simulink model "B_LazoCerrado_PI"  (R2017a)
settings: Solver=FixedStepAuto  StartTime=0.0  StopTime=inf  RelTol=1e-3  EnableMultiTasking=on
libraries: arduinolib x2, simulink x1
settings Model: SimulationMode=external  ExtModeTrigDuration=2  Creator=pablo  LastModifiedBy=pablo
settings OptimizationCC: PassReuseOutputArgsAs=Individual arguments  MaxStackSize=64
settings DebuggingCC: ParameterTunabilityLossMsg=error
settings HardwareCC: ProdBitPerInt=16  ProdBitPerPointer=16  ProdBitPerSizeT=16  ProdBitPerPtrDiffT=16  ProdLargestAtomicFloat=None  ProdWordSize=8  ProdHWDeviceType=Atmel->AVR
settings SFSimCC: MATLABDynamicMemAlloc=off
settings RTWCC: SystemTargetFile=ert.tlc  HardwareBoard=Arduino Uno  TLCOptions=-aInlineSetEventsForThisBaseRateFcn=TLC_FALSE -aSuppressMultiTaskScheduler=TLC_FALSE -aRateBasedStepFcn=1  TemplateMakefile=ert_default_tmf  Description=Embedded Coder  GenerateReport=on  Toolchain=Arduino AVR  BuildConfiguration=Faster Runs  IncludeHyperlinkInReport=on  LaunchReport=on  GenerateTraceInfo=on  GenerateTraceReport=on  GenerateTraceReportSl=on  GenerateTraceReportSf=on  GenerateTraceReportEml=on
settings CodeAppCC: ForceParamTrailComments=on  IgnoreCustomStorageClasses=off  OperatorAnnotations=on  SimulinkDataObjDesc=on  SFDataObjDesc=on  MATLABFcnDesc=on  InsertBlockDesc=on  MATLABSourceComments=on
settings ERTTargetCC: SupportContinuousTime=on  SupportVariableSizeSignals=on

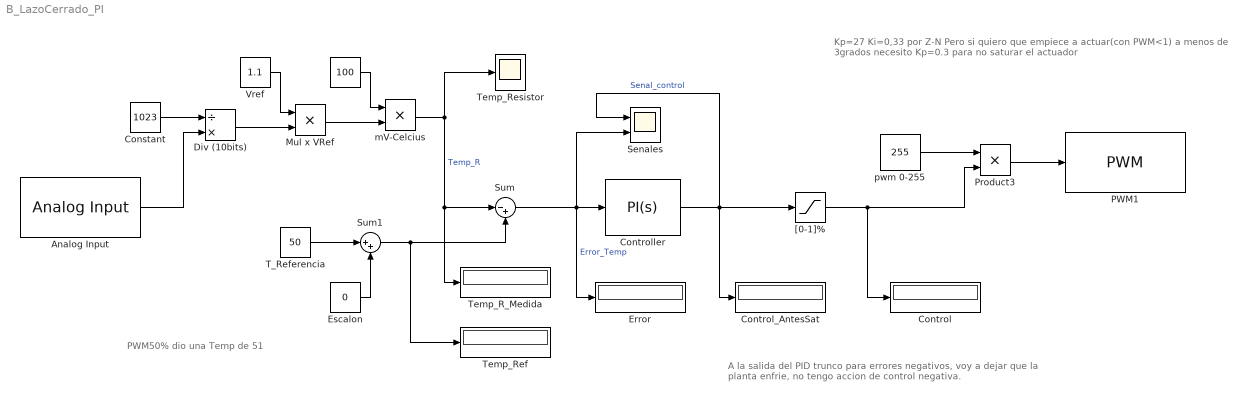
== system B_LazoCerrado_PI ==
  note: PWM50% dio una Temp de 51
  note: Kp=27 Ki=0,33 por Z-N
      | Pero si quiero que empiece a actuar(con PWM<1)
      | a menos de 3grados necesito Kp=0.3
      | para no saturar el actuador
  note: A la salida del PID trunco para errores negativos,
      | voy a dejar que la planta enfrie, no tengo accion de control negativa.
  " " : Constant  Value=100
  " Controller" : simulink/Continuous/PID Controller  Controller=PI  TimeDomain=Continuous-time  SampleTime=-1  IntegratorMethod=Forward Euler  FilterMethod=Forward Euler  Form=Parallel  UseFilter=on  ControllerParametersSource=internal  P=0.1  I=0.0001  D=0  N=100  InitialConditionSource=internal  InitialConditionForIntegrator=0  InitialConditionForFilter=0  ExternalReset=none  LimitOutput=on  UpperSaturationLimit=inf  LowerSaturationLimit=0  LinearizeAsGain=on  AntiWindupMode=none  Kb=1  TrackingMode=off  Kt=1  PParamMin=[]  PParamMax=[]  IParamMin=[]  IParamMax=[]  DParamMin=[]  DParamMax=[]  NParamMin=[]  NParamMax=[]  KbParamMin=[]  KbParamMax=[]  KtParamMin=[]  KtParamMax=[]  POutMin=[]  POutMax=[]  IOutMin=[]  IOutMax=[]  DOutMin=[]  DOutMax=[]  NOutMin=[]  NOutMax=[]  KbOutMin=[]  KbOutMax=[]  KtOutMin=[]  KtOutMax=[]  IntegratorOutMin=[]  IntegratorOutMax=[]  FilterOutMin=[]  FilterOutMax=[]  SumOutMin=[]  SumOutMax=[]  SumI1OutMin=[]  SumI1OutMax=[]  SumI2OutMin=[]  SumI2OutMax=[]  SumI3OutMin=[]  SumI3OutMax=[]  SumDOutMin=[]  SumDOutMax=[]  SaturationOutMin=[]  SaturationOutMax=[]  IntegratorContinuousStateAttributes=''  IntegratorStateMustResolveToSignalObject=off  IntegratorRTWStateStorageClass=Auto  FilterContinuousStateAttributes=''  FilterStateMustResolveToSignalObject=off  FilterRTWStateStorageClass=Auto  DifferentiatorICPrevScaledInput=0  DifferentiatorOutMin=[]  DifferentiatorOutMax=[]  InitialConditionSetting=State (most efficient)
  " Escalon " : Constant  Value=0
  " T_Referencia " : Constant  Value=50
  " Vref " : Constant  Value=1.1
  " pwm 0-255" : Constant  Value=255
  Analog Input : arduinolib/Analog Input  pinNumber=0  sampleTime=0.1  blockPlatform=arduino
  Constant : Constant  Value=1023
  Control : Display
      settings: Decimation=2
  Control_AntesSat : Display
      settings: Decimation=2
  Div (10bits) : Product  Inputs=/*
  Error : Display
      settings: Decimation=2
  Mul x VRef : Product
  PWM1 : arduinolib/PWM  pinNumber=5  blockPlatform=arduino
  Product3 : Product
  "Senales " : Scope  NumInputPorts=2
  Sum : Sum  Inputs=|-+
  Sum1 : Sum  Inputs=|++
  Temp_R_Medida : Display
      settings: Decimation=2
  Temp_Ref : Display
      settings: Format=decimal (Stored Integer)  Decimation=2
  Temp_Resistor : Scope
  "[0-1]%" : Saturate  UpperLimit=1  LowerLimit=0
  mV-Celcius : Product
  wires:
  Div (10bits)/1 -> Mul x VRef/2
  Analog Input/1 -> Div (10bits)/2
  Constant/1 -> Div (10bits)/1
  " Vref "/1 -> Mul x VRef/1
  Mul x VRef/1 -> mV-Celcius/2
  " "/1 -> mV-Celcius/1
  mV-Celcius/1 -> Temp_Resistor/1, Sum/1, Temp_R_Medida/1  "Temp_R"
  Sum1/1 -> Sum/2, Temp_Ref/1
  " Controller"/1 -> "Senales "/1, "[0-1]%"/1, Control_AntesSat/1  "Senal_control"
  Sum/1 -> " Controller"/1, "Senales "/2, Error/1  "Error_Temp"
  "[0-1]%"/1 -> Control/1, Product3/2
  " pwm 0-255"/1 -> Product3/1
  Product3/1 -> PWM1/1
  " Escalon "/1 -> Sum1/2
  " T_Referencia "/1 -> Sum1/1
